simulink model "stateflow_project"  (R2020a)
settings: Solver=VariableStepAuto  StartTime=0.0  StopTime=inf  RelTol=1e-3
settings Model: EnablePacing=on  PacingRate=40  Creator=joshi  LastModifiedBy=joshi

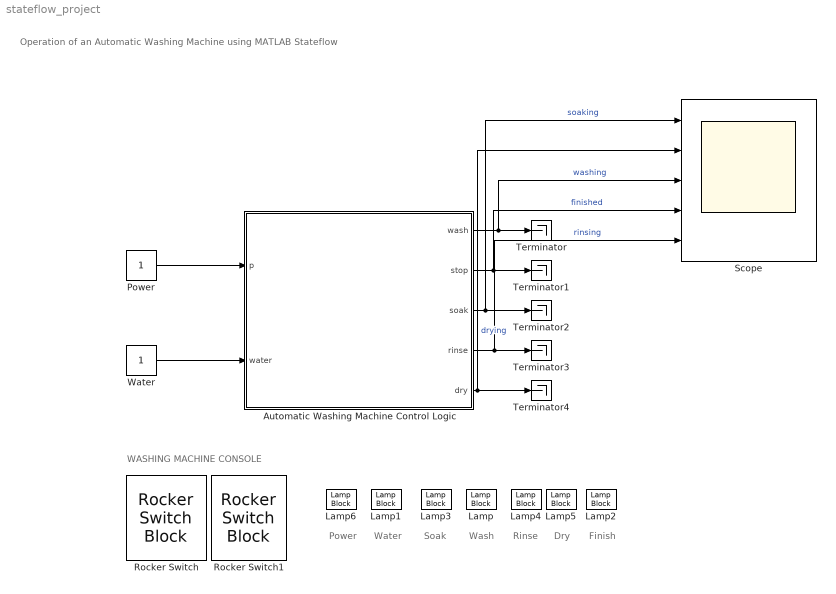
== system stateflow_project ==
  note: Operation of an Automatic Washing Machine using MATLAB Stateflow
  note: Wash
  note: WASHING MACHINE CONSOLE
  note: Water
  note: Finish
  note: Soak
  note: Rinse
  note: Dry
  note: Power
  Automatic Washing Machine Control Logic : Stateflow chart  TreatAsAtomicUnit=on
  Lamp{,1..6} (7 alike) : LampBlock  LabelPosition=Hide
  Power : Constant
  Rocker Switch : RockerSwitchBlock  LabelPosition=Bottom
      settings: Values={{'Off', 'On'}, [0 1]}
  Rocker Switch1 : RockerSwitchBlock  LabelPosition=Bottom
      settings: Values={{'Off', 'On'}, [0 1]}
  Scope : Scope  NumInputPorts=5
  Terminator{,1..4} (5 alike) : Terminator
  Water : Constant
  wires:
  Power/1 -> Automatic Washing Machine Control Logic/1(p)
  Water/1 -> Automatic Washing Machine Control Logic/2(water)
  Automatic Washing Machine Control Logic/1(wash) -> Scope/3, Terminator/1  "washing"
  Automatic Washing Machine Control Logic/2(stop) -> Scope/4, Terminator1/1  "finished"
  Automatic Washing Machine Control Logic/3(soak) -> Scope/1, Terminator2/1  "soaking"
  Automatic Washing Machine Control Logic/4(rinse) -> Terminator3/1, Scope/5  "rinsing"
  Automatic Washing Machine Control Logic/5(dry) -> Scope/2, Terminator4/1  "drying"

== stateflow chart stateflow_project/Automatic Washing Machine Control Logic ==
  state Power
  state Off
  state ON
  state Water_supply
    entry: w=1;
    exit: w=0
  state a
  state Soaking
    entry: soak=1;
    exit: soak=0;
  state b
  state Washing
    entry: wash=1;
    exit: wash=0;
  state c
  state Rinsing
    entry: rinse=1;
    exit: rinse=0;
  state d
  state Drying
    entry: dry=1;
    exit: dry=0;
  state e
  state Stop
    entry: stop=0;
    exit: stop=1;
  (junction 96) -> (junction 59)
  Off -> (junction 96) [order 2] : [p==1 && water==1]
  (junction 59) -> (junction 103)
  (junction 87) -> (junction 59)
  (junction 103) -> (junction 105)
  (junction 105) -> Power
  (default) -> Power
  Power -> Off [order 1] : [p==0]
  Power -> ON [order 2] : [p==1]
  ON -> Off [order 1] : [water==0]
  Off -> ON [order 1] : [water==1&& p==1]
  ON -> Water_supply [order 2] : [water>0]
  Water_supply -> a [order 1] : [p==0]
  a -> Water_supply : [p==1]
  Water_supply -> Soaking [order 2]
  Soaking -> b [order 2] : [p==0]
  b -> Soaking : [p==1 && water==1]
  Soaking -> Washing [order 1] : after(200,sec)
  Washing -> c [order 2] : [p==0]
  c -> Washing : [p==1 && water==1]
  Washing -> Rinsing [order 1] : after(100,sec)
  Rinsing -> d [order 2] : [p==0]
  d -> Rinsing : [p==1 && water==1]
  Rinsing -> Drying [order 1] : after(20,sec)
  Drying -> e [order 2] : [p==0]
  e -> Drying : [p==1 && water==1]
  Drying -> Stop [order 1] : after(50,sec)
  Stop -> (junction 87)
  data: p input; water input; wash output; stop output; soak output; rinse output; dry output; w local
